simulink model "Copy_of_u_perf_FlightModel"  (R2018b)
settings: Solver=VariableStepAuto  StartTime=0.0  StopTime=10.0  RelTol=1e-3
libraries: cstblocks x7
settings Model: Creator=nikovertovec  LastModifiedBy=nikovertovec
settings DataIOCC: SaveFinalState=on  SaveState=on

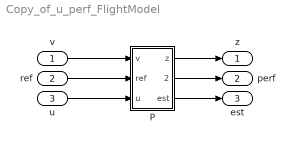
== system Copy_of_u_perf_FlightModel ==
  v : Inport
  ref : Inport  Port=2
  u : Inport  Port=3
  P : Subsystem
  z : Outport
  perf : Outport  Port=2
  est : Outport  Port=3
  wires:
  v/1 -> P/1(v)
  ref/1 -> P/2(ref)
  u/1 -> P/3(u)
  P/1(z) -> z/1
  P/2(perf) -> perf/1
  P/3(est) -> est/1

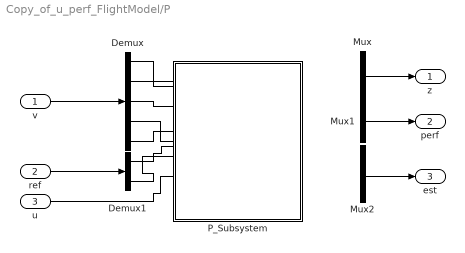
== system Copy_of_u_perf_FlightModel/P ==
  v : Inport
  ref : Inport  Port=2
  u : Inport  Port=3
  Demux : Demux  Outputs=5
  Demux1 : Demux  Outputs=2
  Mux : Mux  Inputs=3
  Mux1 : Mux  Inputs=3
  Mux2 : Mux
  P_Subsystem : Subsystem
  z : Outport
  perf : Outport  Port=2
  est : Outport  Port=3
  wires:
  Mux2/1 -> est/1
  Demux/1 -> ?
  ref/1 -> Demux1/1
  Demux1/1 -> ?
  ? -> Mux2/2
  ? -> Mux2/1
  Demux1/2 -> ?
  ? -> Mux1/2
  Demux/5 -> ?
  Mux1/1 -> perf/1
  Demux/4 -> ?
  Demux/3 -> ?
  ? -> Mux/3
  ? -> Mux/2
  Mux/1 -> z/1
  ? -> Mux/1
  ? -> Mux1/1
  Demux/2 -> ?
  u/1 -> ?
  v/1 -> Demux/1
  ? -> Mux2/3
  ? -> Mux2/4
  ? -> Mux1/3

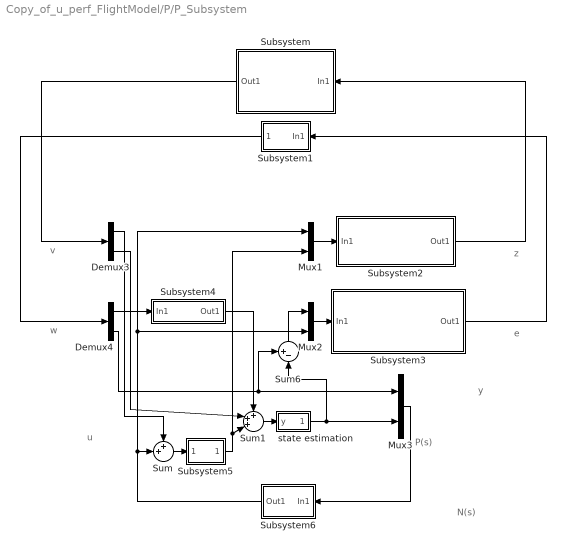
== system Copy_of_u_perf_FlightModel/P/P_Subsystem ==
  note: N(s)
  note: w
  note: P(s)
  note: v
  note: u
  note: y
  note: e
  note: z
  Demux3 : Demux  Outputs=2
  Demux4 : Demux  Outputs=2
  Mux1 : Mux  Inputs=2
  Mux2 : Mux  Inputs=2
  Mux3 : Mux  Inputs=2
  Subsystem : Subsystem
      mask Display: image('/Users/nikovertovec/Documents/MATLAB/Advance Topics in Control/Project/IconImages/delta.png');
  Subsystem1 : Subsystem
      mask Display: image('/Users/nikovertovec/Documents/MATLAB/Advance Topics in Control/Project/IconImages/Delta_p.png');
  Subsystem2 : Subsystem
      mask Display: image('/Users/nikovertovec/Documents/MATLAB/Advance Topics in Control/Project/IconImages/W_delta.png');
  Subsystem3 : Subsystem
      mask Display: image('/Users/nikovertovec/Documents/MATLAB/Advance Topics in Control/Project/IconImages/Wp.png');
  Subsystem4 : Subsystem
      mask Display: image('/Users/nikovertovec/Documents/MATLAB/Advance Topics in Control/Project/IconImages/W_sensorNoise.png');
  Subsystem5 : Subsystem
      mask Display: image('/Users/nikovertovec/Documents/MATLAB/Advance Topics in Control/Project/IconImages/G.png');
  Subsystem6 : Subsystem
      mask Display: image('/Users/nikovertovec/Documents/MATLAB/Advance Topics in Control/Project/IconImages/K.png');
  Sum : Sum  Inputs=++|  OutMin=0  OutMax=1
  Sum1 : Sum  Inputs=+++|  OutMin=0  OutMax=1
  Sum6 : Sum  Inputs=+-|  OutMin=0  OutMax=1
  state estimation : Subsystem
      mask Display: image('/Users/nikovertovec/Documents/MATLAB/Advance Topics in Control/Project/IconImages/Est.png');
  wires:
  Demux3/2 -> Sum1/2
  Demux3/1 -> Sum/1
  Demux4/2 -> Sum6/1, Mux3/1
  Sum1/1 -> state estimation/1(y)
  state estimation/1("x_est ") -> Mux3/2, Sum6/2
  Sum6/1 -> Mux2/1
  Subsystem/1(Out1) -> Demux3/1
  Subsystem1/1(Out1) -> Demux4/1
  Mux1/1 -> Subsystem2/1(In1)
  Subsystem2/1(Out1) -> Subsystem/1(In1)
  Mux2/1 -> Subsystem3/1(In1)
  Subsystem3/1(Out1) -> Subsystem1/1(In1)
  Demux4/1 -> Subsystem4/1(In1)
  Subsystem4/1(Out1) -> Sum1/1
  Subsystem5/1(Out1) -> Mux1/2, Sum1/3
  Sum/1 -> Subsystem5/1(In1)
  Subsystem6/1(Out1) -> Sum/2, Mux1/1, Mux2/2
  Mux3/1 -> Subsystem6/1(In1)

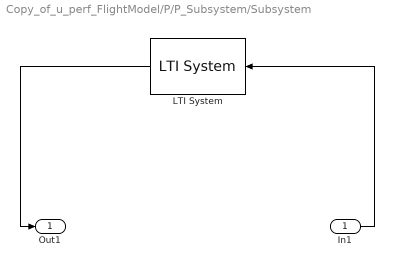
== system Copy_of_u_perf_FlightModel/P/P_Subsystem/Subsystem ==
  In1 : Inport
  LTI System : cstblocks/LTI System  sys=tf(1,[1 1])  IC=[]  mask(LTI Block){}
      mask Display: image('/Users/nikovertovec/Documents/MATLAB/Advance Topics in Control/Project/IconImages/delta.png');
  Out1 : Outport
  wires:
  In1/1 -> LTI System/1
  LTI System/1 -> Out1/1

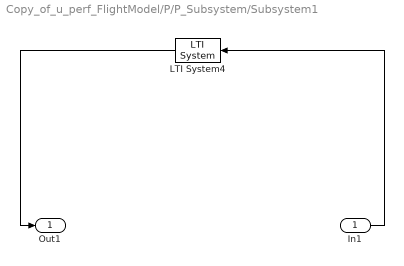
== system Copy_of_u_perf_FlightModel/P/P_Subsystem/Subsystem1 ==
  In1 : Inport
  LTI System4 : cstblocks/LTI System  sys=tf(1,[1 1])  IC=[]  mask(LTI Block){}
      mask Display: image('/Users/nikovertovec/Documents/MATLAB/Advance Topics in Control/Project/IconImages/Delta_p.png');
  Out1 : Outport
  wires:
  LTI System4/1 -> Out1/1
  In1/1 -> LTI System4/1

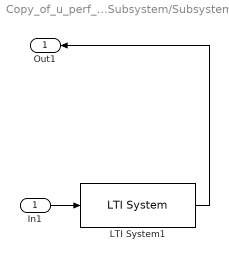
== system Copy_of_u_perf_FlightModel/P/P_Subsystem/Subsystem2 ==
  In1 : Inport
  LTI System1 : cstblocks/LTI System  sys=W_delta  IC=[]  mask(LTI Block){}
      mask Display: image('/Users/nikovertovec/Documents/MATLAB/Advance Topics in Control/Project/IconImages/W_delta.png');
  Out1 : Outport
  wires:
  LTI System1/1 -> Out1/1
  In1/1 -> LTI System1/1

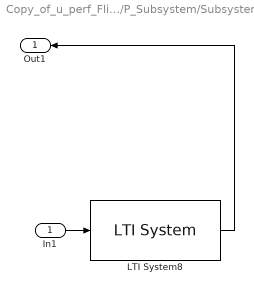
== system Copy_of_u_perf_FlightModel/P/P_Subsystem/Subsystem3 ==
  In1 : Inport
  LTI System8 : cstblocks/LTI System  sys=Wp  IC=[]  mask(LTI Block){}
      mask Display: image('/Users/nikovertovec/Documents/MATLAB/Advance Topics in Control/Project/IconImages/Wp.png');
  Out1 : Outport
  wires:
  LTI System8/1 -> Out1/1
  In1/1 -> LTI System8/1

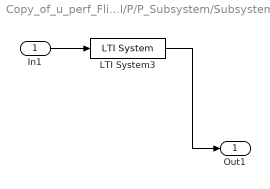
== system Copy_of_u_perf_FlightModel/P/P_Subsystem/Subsystem4 ==
  In1 : Inport
  LTI System3 : cstblocks/LTI System  sys=W_sensorNoise  IC=[]  mask(LTI Block){}
      mask Display: image('/Users/nikovertovec/Documents/MATLAB/Advance Topics in Control/Project/IconImages/W_sensorNoise.png');
  Out1 : Outport
  wires:
  LTI System3/1 -> Out1/1
  In1/1 -> LTI System3/1

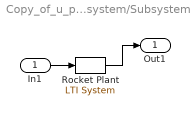
== system Copy_of_u_perf_FlightModel/P/P_Subsystem/Subsystem5 ==
  In1 : Inport
  Rocket Plant : cstblocks/LTI System  sys=G  IC=[]  mask(LTI Block){}
      mask Display: image('/Users/nikovertovec/Documents/MATLAB/Advance Topics in Control/Project/IconImages/G.png');
  Out1 : Outport
  wires:
  Rocket Plant/1 -> Out1/1
  In1/1 -> Rocket Plant/1

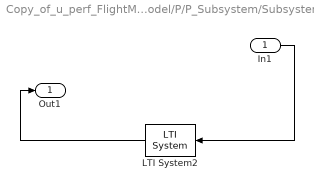
== system Copy_of_u_perf_FlightModel/P/P_Subsystem/Subsystem6 ==
  In1 : Inport
  LTI System2 : cstblocks/LTI System  sys=tf(1,[1 1])  IC=[]  mask(LTI Block){}
      mask Display: image('/Users/nikovertovec/Documents/MATLAB/Advance Topics in Control/Project/IconImages/K.png');
  Out1 : Outport
  wires:
  In1/1 -> LTI System2/1
  LTI System2/1 -> Out1/1

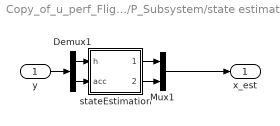
== system Copy_of_u_perf_FlightModel/P/P_Subsystem/state estimation ==
  y : Inport
  Demux1 : Demux  Outputs=2
  Mux1 : Mux  Inputs=2
  stateEstimation : Subsystem
  "x_est " : Outport
  wires:
  y/1 -> Demux1/1
  stateEstimation/2(v_est) -> Mux1/2
  stateEstimation/1(h_est) -> Mux1/1
  Demux1/2 -> stateEstimation/2(acc)
  Mux1/1 -> "x_est "/1
  Demux1/1 -> stateEstimation/1(h)

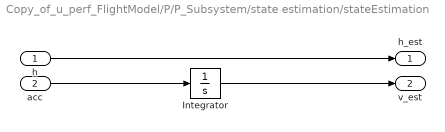
== system Copy_of_u_perf_FlightModel/P/P_Subsystem/state estimation/stateEstimation ==
  h : Inport
  acc : Inport  Port=2
  Integrator : Integrator
  h_est : Outport
  v_est : Outport  Port=2
  wires:
  acc/1 -> Integrator/1
  h/1 -> h_est/1
  Integrator/1 -> v_est/1
